simulink model "DEC_DIP_p2014"  (R2013b)
settings: Solver=ode5  StartTime=0.01  StopTime=sim_time  FixedStep=0.01  MaxStep=0.001  RelTol=1e-6  AbsTol=1e-6
undefined symbols (not defined in the file or in its folder): Ankle_Gain, body_mgh, dt_ankle, dt_hip, g, h_COM_L, h_COM_T, Hip_Gain, J_B, J_L, J_T, Kd_A_p, Kd_H_p, Kp_A_p, Kp_H_p, l_L, l_T, m_B, m_L, m_T, mgh_B, mgh_T, pp, th_grav_bs, th_grav_ts, th_vfs, trunk_mgh, wf_grav_bs, wf_grav_ts, wf_T_ext_A, wf_T_ext_H, wf_Trans, wf_vfs
settings Model: ExtModeAutoUpdateStatusClock=off  Creator=thomasmergner  LastModifiedBy=lorenz
settings SolverCC: InitialStep=0.001  AutoInsertRateTranBlk=on
settings DataIOCC: LimitDataPoints=off  SignalLoggingSaveFormat=ModelDataLogs  SaveOutput=off  SignalLogging=off  DSMLogging=off  SaveTime=off  ReturnWorkspaceOutputs=on
settings OptimizationCC: BlockReduction=off  BooleanDataType=off  ExpressionDepthLimit=2147483647  InitFltsAndDblsToZero=on
settings DebuggingCC: SaveWithParameterizedLinksMsg=none  SignalResolutionControl=TryResolveAllWithWarning  SolverPrmCheckMsg=none  InheritedTsInSrcMsg=none  MultiTaskDSMMsg=warning  MultiTaskCondExecSysMsg=none  FcnCallInpInsideContextMsg=UseLocalSettings  StateNameClashWarn=warning
settings HardwareCC: TargetUnknown=on
settings RTWCC: IncludeERTFirstTime=on
settings GRTTargetCC: TargetFcnLib=ansi_tfl_tmw.mat  CombineOutputUpdateFcns=off  GRTInterface=on

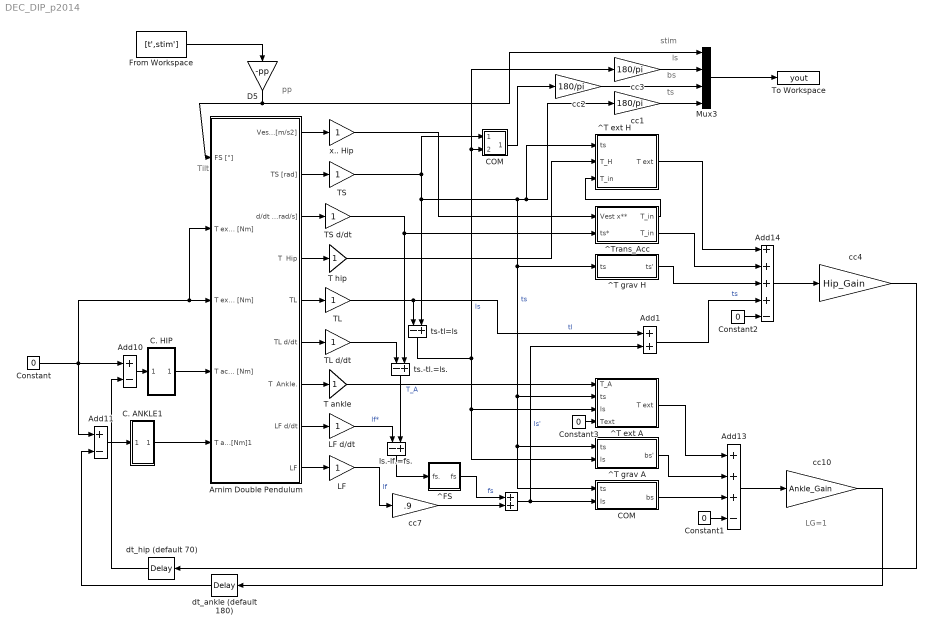
== system DEC_DIP_p2014 ==
  note: Tilt
  note: pp
  note: stim
  note: ls
  note: bs
  note: ts
  note: LG=1
  " " : Sum
  Add1 : Sum
  Add10 : Sum  Inputs=+-
  Add11 : Sum  Inputs=+-
  Add13 : Sum  Inputs=+++-
  Add14 : Sum  Inputs=++++-
  Arnim Double Pendulum : Subsystem
  C. ANKLE1 : Subsystem
  C. HIP : Subsystem
  COM : Subsystem
  "COM " : Subsystem
  Constant{,1..3} (4 alike) : Constant  Value=0
  D5 : Gain  Gain=-pp  SaturateOnIntegerOverflow=on  OutDataTypeStr=Inherit: Same as input  ParamDataTypeStr=Inherit: Same as input
  From Workspace : FromWorkspace  VariableName=[t',stim']
  "LF " : Gain
  LF d/dt : Gain
  Mux3 : Mux
  T ankle : Gain
  T hip : Gain
  TL : Gain
  TL d/dt : Gain
  TS : Gain
  TS d/dt : Gain
  To Workspace : ToWorkspace  VariableName=yout
  ^FS : Subsystem
  ^T ext A : Subsystem
  ^T ext H : Subsystem
  ^T grav A : Subsystem
  ^T grav H : Subsystem
  ^Trans_Acc : Subsystem
  cc1 : Gain  Gain=180/pi
  cc10 : Gain  Gain=Ankle_Gain
  cc2 : Gain  Gain=180/pi
  cc3 : Gain  Gain=180/pi
  cc4 : Gain  Gain=Hip_Gain
  cc7 : Gain  Gain=.9
  dt_ankle (default 180) : TransportDelay  DelayTime=dt_ankle
  dt_hip (default 70) : TransportDelay  DelayTime=dt_hip
  ls.-lf.=fs. : Sum  Inputs=-+
  ts-tl=ls : Sum  Inputs=-+
  ts.-tl.=ls. : Sum  Inputs=-+
  x.. Hip : Gain
  wires:
  Add11/1 -> C. ANKLE1/1(C_)
  Add10/1 -> C. HIP/1("C_   ")
  Arnim Double Pendulum/9(LF) -> "LF "/1
  Arnim Double Pendulum/8(LF d/dt) -> LF d/dt/1
  "LF "/1 -> cc7/1  "lf"
  ls.-lf.=fs./1 -> ^FS/1(fs.)
  TL/1 -> ts-tl=ls/1, Add1/1  "tl"
  Add14/1 -> cc4/1
  ts-tl=ls/1 -> ^T grav A/2(ls), ^T ext A/3(ls), cc3/1, "COM "/2(Is)  "ls"
  Arnim Double Pendulum/4("T  Hip ") -> T hip/1
  TS/1 -> cc1/1, ^T ext H/1(ts), ^T ext A/2(ts), ^T grav A/1(ts), COM/1(ts), ^T grav H/1(ts), ts-tl=ls/2, "COM "/1(ts)  "ts"
  Mux3/1 -> To Workspace/1
  Add13/1 -> cc10/1
  D5/1 -> Arnim Double Pendulum/1(FS [°]), Mux3/1
  From Workspace/1 -> D5/1
  cc4/1 -> dt_hip (default 70)/1
  " "/1 -> COM/2(Is), Add1/2  "ls'"
  cc10/1 -> dt_ankle (default 180)/1
  Arnim Double Pendulum/1(Vest_Acc [m/s2]) -> x.. Hip/1
  x.. Hip/1 -> ^Trans_Acc/1(Vest x**)
  cc3/1 -> Mux3/2
  cc2/1 -> Mux3/3
  cc1/1 -> Mux3/4
  C. HIP/1(Hip) -> Arnim Double Pendulum/4(T act hip [Nm])
  C. ANKLE1/1(" An") -> Arnim Double Pendulum/5(" T act ankle [Nm]1")
  LF d/dt/1 -> ls.-lf.=fs./1  "lf*"
  Arnim Double Pendulum/6(TL d/dt) -> TL d/dt/1
  Arnim Double Pendulum/7(T  Ankle.) -> T ankle/1
  Arnim Double Pendulum/5(TL) -> TL/1
  ts.-tl.=ls./1 -> ls.-lf.=fs./2
  Arnim Double Pendulum/3(d/dt TS[rad/s]) -> TS d/dt/1
  Arnim Double Pendulum/2(TS [rad]) -> TS/1
  TS d/dt/1 -> ts.-tl.=ls./2, ^Trans_Acc/2(ts*)
  TL d/dt/1 -> ts.-tl.=ls./1
  COM/1(bs) -> Add13/3
  T ankle/1 -> ^T ext A/1(T_A)  "T_A"
  ^T grav A/1(bs') -> Add13/2
  ^T grav H/1(ts') -> Add14/3
  T hip/1 -> ^T ext H/2(T_H)
  "COM "/1(bs) -> cc2/1
  dt_ankle (default 180)/1 -> Add11/2
  dt_hip (default 70)/1 -> Add10/2
  ^Trans_Acc/1("T_in ") -> ^T ext H/3(T_in)
  ^FS/1(fs) -> " "/1  "fs"
  cc7/1 -> " "/2
  ^T ext A/1(T ext) -> Add13/1
  Add1/1 -> Add14/4  "ts"
  ^T ext H/1(T ext) -> Add14/1
  ^Trans_Acc/2(T_in) -> Add14/2
  Constant/1 -> Arnim Double Pendulum/2(T ext hip [Nm]), Arnim Double Pendulum/3(T ext ankle [Nm]), Add11/1, Add10/1
  Constant1/1 -> Add13/4
  Constant2/1 -> Add14/5
  Constant3/1 -> ^T ext A/4(Text)

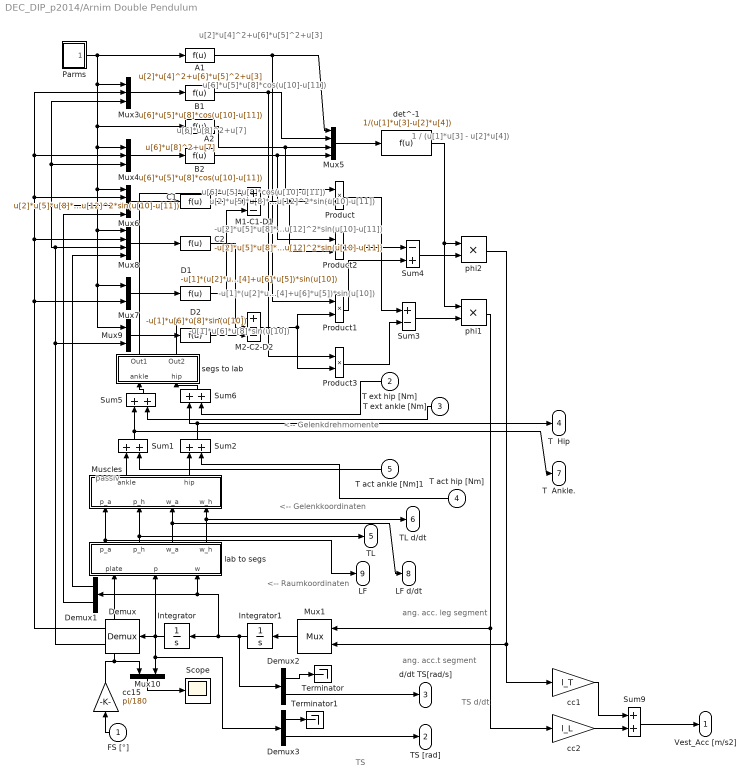
== system DEC_DIP_p2014/Arnim Double Pendulum ==
  note: <-- Gelenkkoordinaten
  note: <-- Gelenkdrehmomente
  note: <-- Raumkoordinaten
  note: ang. acc. leg segment
  note: ang. acc.t segment
  note: u[2]*u[4]^2+u[6]*u[5]^2+u[3]
  note: 1 / (u[1]*u[3] - u[2]*u[4])
  note: u[6]*u[5]*u[8]*cos(u[10]-u[11])
  note: u[6]*u[8]^2+u[7]
  note: u[6]*u[5]*u[8]*cos(u[10]-u[11])
  note: u[2]*u[5]*u[8]*u[12]^2*sin(u[10]-u[11])
  note: -u[2]*u[5]*u[8]*u[12]^2*sin(u[10]-u[11])
  note: -u[1]*(u[2]*u[4]+u[6]*u[5])*sin(u[10])
  note: -u[1]*u[6]*u[8]*sin(u[10])
  note: TS d/dt
  note: TS
  note: passiv
  FS [°] : Inport
  T ext hip [Nm] : Inport  Port=2
  T ext ankle [Nm] : Inport  Port=3
  T act hip [Nm] : Inport  Port=4
  " T act ankle [Nm]1" : Inport  Port=5
  A1 : Fcn  Expr=u[2]*u[4]^2+u[6]*u[5]^2+u[3]
  A2 : Fcn  Expr=u[6]*u[8]^2+u[7]
  B1 : Fcn  Expr=u[6]*u[5]*u[8]*cos(u[10]-u[11])
  B2 : Fcn  Expr=u[6]*u[5]*u[8]*cos(u[10]-u[11])
  C1 : Fcn  Expr=u[2]*u[5]*u[8]*u[12]^2*sin(u[10]-u[11])
  C2 : Fcn  Expr=-u[2]*u[5]*u[8]*u[12]^2*sin(u[10]-u[11])
  D1 : Fcn  Expr=-u[1]*(u[2]*u[4]+u[6]*u[5])*sin(u[10])
  D2 : Fcn  Expr=-u[1]*u[6]*u[8]*sin(u[10])
  Demux{,1..3} (4 alike) : Demux  Outputs=2
  Integrator : Integrator  InitialCondition=[0.0*pi,0.0*pi]
  Integrator1 : Integrator  InitialCondition=[0,0]
  M1-C1-D1 : Sum  Inputs=+--  SaturateOnIntegerOverflow=on  InputSameDT=on  OutDataTypeStr=Inherit: Same as first input
  M2-C2-D2 : Sum  Inputs=+--  SaturateOnIntegerOverflow=on  InputSameDT=on  OutDataTypeStr=Inherit: Same as first input
  Muscles : Subsystem
  Mux{1,7,9..10} (4 alike) : Mux  Inputs=2
  Mux3 : Mux  Inputs=3
  Mux4 : Mux  Inputs=3
  Mux5 : Mux
  Mux6 : Mux
  Mux8 : Mux
  Parms : Subsystem
  Product{,1..3} (4 alike) : Product  SaturateOnIntegerOverflow=on  RndMeth=Zero  InputSameDT=on  OutDataTypeStr=Inherit: Same as first input
  Scope : Scope
      settings: TickLabels=on  YMin=-0.0005  YMax=0.0045
  Sum{1..2,5..6,9} (5 alike) : Sum  SaturateOnIntegerOverflow=on  InputSameDT=on  OutDataTypeStr=Inherit: Same as first input
  Sum3 : Sum  Inputs=+-  SaturateOnIntegerOverflow=on  InputSameDT=on  OutDataTypeStr=Inherit: Same as first input
  Sum4 : Sum  Inputs=-+  SaturateOnIntegerOverflow=on  InputSameDT=on  OutDataTypeStr=Inherit: Same as first input
  Terminator : Terminator
  Terminator1 : Terminator
  cc1 : Gain  Gain=l_T
  cc15 : Gain  Gain=pi/180
  cc2 : Gain  Gain=l_L
  det^-1 : Fcn  Expr=1/(u[1]*u[3]-u[2]*u[4])
  lab to segs : Subsystem
  phi1 : Product  SaturateOnIntegerOverflow=on  RndMeth=Zero  InputSameDT=on  OutDataTypeStr=Inherit: Same as first input
  phi2 : Product  SaturateOnIntegerOverflow=on  RndMeth=Zero  InputSameDT=on  OutDataTypeStr=Inherit: Same as first input
  segs to lab : Subsystem
  Vest_Acc [m/s2] : Outport  InitialOutput=0
  TS [rad] : Outport  Port=2  InitialOutput=0
  d/dt TS[rad/s] : Outport  Port=3  InitialOutput=0
  "T  Hip " : Outport  Port=4  InitialOutput=0
  TL : Outport  Port=5  InitialOutput=0
  TL d/dt : Outport  Port=6  InitialOutput=0
  T  Ankle. : Outport  Port=7  InitialOutput=0
  LF d/dt : Outport  Port=8  InitialOutput=0
  LF : Outport  Port=9  InitialOutput=0
  wires:
  Mux4/1 -> B2/1
  Mux3/1 -> B1/1
  Mux6/1 -> C1/1
  Mux8/1 -> C2/1
  Mux9/1 -> D2/1
  Mux7/1 -> D1/1
  C1/1 -> M1-C1-D1/2
  C2/1 -> M2-C2-D2/2
  D1/1 -> M1-C1-D1/3
  D2/1 -> M2-C2-D2/3
  Parms/1(Out1) -> Mux3/1, A2/1, Mux4/1, Mux9/1, Mux7/1, Mux8/1, Mux6/1, A1/1
  A2/1 -> Mux5/3, Product/1
  M1-C1-D1/1 -> Product/2, Product2/2
  B2/1 -> Mux5/4, Product2/1
  M2-C2-D2/1 -> Product1/2, Product3/2
  A1/1 -> Mux5/1, Product1/1
  B1/1 -> Mux5/2, Product3/1
  Mux5/1 -> det^-1/1
  Product2/1 -> Sum4/1
  Product1/1 -> Sum4/2
  Product3/1 -> Sum3/2
  Product/1 -> Sum3/1
  Sum4/1 -> phi2/2
  Sum3/1 -> phi1/2
  det^-1/1 -> phi2/1, phi1/1
  phi2/1 -> Mux1/2, cc1/1
  Demux/1 -> Mux3/2, Mux4/2, Mux6/2, Mux8/2, Mux7/2
  Demux/2 -> Mux3/3, Mux4/3, Mux6/3, Mux8/3, Mux9/2
  Demux1/1 -> Mux8/4
  Demux1/2 -> Mux6/4
  segs to lab/1(Out1) -> M1-C1-D1/1
  segs to lab/2(Out2) -> M2-C2-D2/1
  Mux1/1 -> Integrator1/1
  Integrator1/1 -> Integrator/1, Demux1/1, lab to segs/3(w), Demux2/1
  Integrator/1 -> Mux10/2, Demux3/1, Demux/1, lab to segs/2(p)
  lab to segs/1(p_a) -> Muscles/1(p_a), LF/1
  lab to segs/2(p_h) -> Muscles/2(p_h), TL/1
  lab to segs/4(w_h) -> Muscles/4(w_h), TL d/dt/1
  lab to segs/3(w_a) -> Muscles/3(w_a), LF d/dt/1
  FS [°]/1 -> cc15/1
  Mux10/1 -> Scope/1
  phi1/1 -> Mux1/1, cc2/1
  " T act ankle [Nm]1"/1 -> Sum1/2
  T act hip [Nm]/1 -> Sum2/2
  Demux2/2 -> d/dt TS[rad/s]/1
  Demux3/2 -> TS [rad]/1
  Sum5/1 -> segs to lab/1(ankle)
  Sum6/1 -> segs to lab/2(hip)
  Sum1/1 -> Sum5/1, T  Ankle./1
  Sum2/1 -> Sum6/1, "T  Hip "/1
  Muscles/1(ankle) -> Sum1/1
  Muscles/2(hip) -> Sum2/1
  cc15/1 -> lab to segs/1(plate), Mux10/1
  T ext hip [Nm]/1 -> Sum6/2
  T ext ankle [Nm]/1 -> Sum5/2
  cc2/1 -> Sum9/2
  Sum9/1 -> Vest_Acc [m/s2]/1
  cc1/1 -> Sum9/1
  Demux2/1 -> Terminator/1
  Demux3/1 -> Terminator1/1

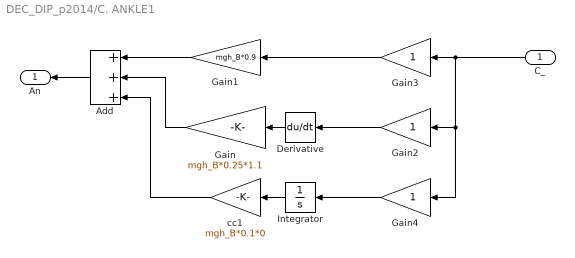
== system DEC_DIP_p2014/C. ANKLE1 ==
  C_ : Inport
  Add : Sum  Inputs=+++
  Derivative : Derivative
  Gain : Gain  Gain=mgh_B*0.25*1.1
  Gain1 : Gain  Gain=mgh_B*0.9
  Gain2 : Gain
  Gain3 : Gain
  Gain4 : Gain
  Integrator : Integrator
  cc1 : Gain  Gain=mgh_B*0.1*0
  " An" : Outport
  wires:
  Derivative/1 -> Gain/1
  Gain/1 -> Add/2
  Gain1/1 -> Add/1
  cc1/1 -> Add/3
  Integrator/1 -> cc1/1
  C_/1 -> Gain2/1, Gain4/1, Gain3/1
  Gain2/1 -> Derivative/1
  Gain3/1 -> Gain1/1
  Gain4/1 -> Integrator/1
  Add/1 -> " An"/1

== system DEC_DIP_p2014/C. HIP ==
  "C_   " : Inport
  Add : Sum  Inputs=+++
  Derivative : Derivative
  Gain : Gain  Gain=mgh_T/4*0.7
  Gain1 : Gain  Gain=mgh_T*0.8
  Gain2 : Gain
  Gain3 : Gain
  Gain4 : Gain
  Integrator : Integrator
  cc2 : Gain  Gain=mgh_T*0.1*0
  Hip : Outport
  wires:
  Add/1 -> Hip/1
  Derivative/1 -> Gain/1
  Gain/1 -> Add/2
  Gain1/1 -> Add/1
  cc2/1 -> Add/3
  Integrator/1 -> cc2/1
  "C_   "/1 -> Gain2/1, Gain3/1, Gain4/1
  Gain2/1 -> Integrator/1
  Gain3/1 -> Derivative/1
  Gain4/1 -> Gain1/1

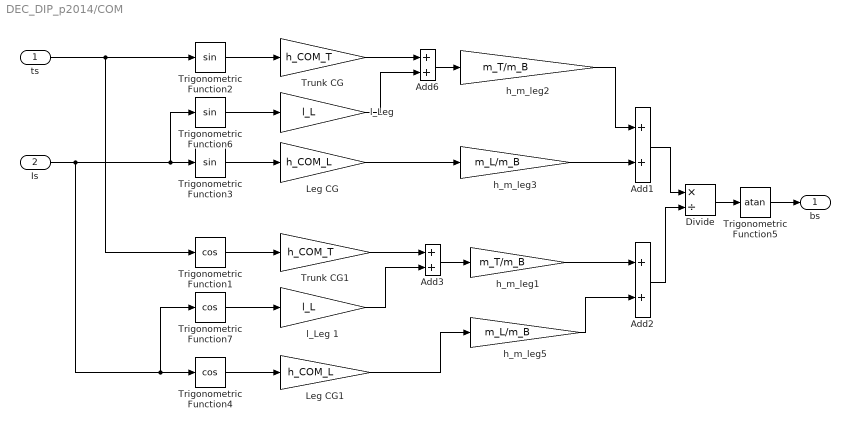
== system DEC_DIP_p2014/COM ==
  ts : Inport
  Is : Inport  Port=2
  Add{1..3,6} (4 alike) : Sum
  Divide : Product  Inputs=*/
  Leg CG : Gain  Gain=h_COM_L
  Leg CG1 : Gain  Gain=h_COM_L
  Trigonometric Function1 : Trigonometry  Operator=cos
  Trigonometric Function2 : Trigonometry
  Trigonometric Function3 : Trigonometry
  Trigonometric Function4 : Trigonometry  Operator=cos
  Trigonometric Function5 : Trigonometry  Operator=atan
  Trigonometric Function6 : Trigonometry
  Trigonometric Function7 : Trigonometry  Operator=cos
  Trunk CG : Gain  Gain=h_COM_T
  Trunk CG1 : Gain  Gain=h_COM_T
  h_m_leg1 : Gain  Gain=m_T/m_B
  h_m_leg2 : Gain  Gain=m_T/m_B
  h_m_leg3 : Gain  Gain=m_L/m_B
  h_m_leg5 : Gain  Gain=m_L/m_B
  "l_Leg " : Gain  Gain=l_L
  l_Leg 1 : Gain  Gain=l_L
  bs : Outport
  wires:
  ts/1 -> Trigonometric Function1/1, Trigonometric Function2/1
  Trigonometric Function2/1 -> Trunk CG/1
  Trigonometric Function3/1 -> Leg CG/1
  Is/1 -> Trigonometric Function3/1, Trigonometric Function6/1, Trigonometric Function4/1, Trigonometric Function7/1
  Trunk CG/1 -> Add6/1
  h_m_leg3/1 -> Add1/2
  Add6/1 -> h_m_leg2/1
  "l_Leg "/1 -> Add6/2
  Trigonometric Function1/1 -> Trunk CG1/1
  Trigonometric Function4/1 -> Leg CG1/1
  Trunk CG1/1 -> Add3/1
  Leg CG1/1 -> h_m_leg5/1
  h_m_leg1/1 -> Add2/1
  h_m_leg5/1 -> Add2/2
  Add3/1 -> h_m_leg1/1
  Add1/1 -> Divide/1
  Divide/1 -> Trigonometric Function5/1
  Trigonometric Function5/1 -> bs/1
  Leg CG/1 -> h_m_leg3/1
  h_m_leg2/1 -> Add1/1
  Add2/1 -> Divide/2
  Trigonometric Function6/1 -> "l_Leg "/1
  Trigonometric Function7/1 -> l_Leg 1/1
  l_Leg 1/1 -> Add3/2

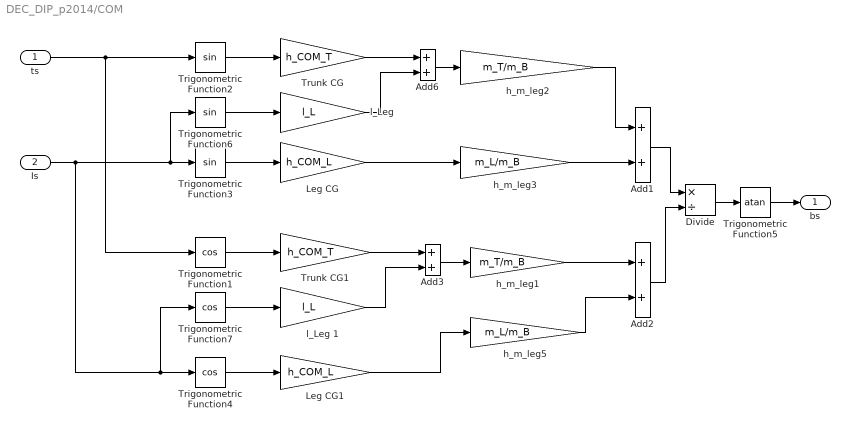
== system DEC_DIP_p2014/COM  ==
  ts : Inport
  Is : Inport  Port=2
  Add{1..3,6} (4 alike) : Sum
  Divide : Product  Inputs=*/
  Leg CG : Gain  Gain=h_COM_L
  Leg CG1 : Gain  Gain=h_COM_L
  Trigonometric Function1 : Trigonometry  Operator=cos
  Trigonometric Function2 : Trigonometry
  Trigonometric Function3 : Trigonometry
  Trigonometric Function4 : Trigonometry  Operator=cos
  Trigonometric Function5 : Trigonometry  Operator=atan
  Trigonometric Function6 : Trigonometry
  Trigonometric Function7 : Trigonometry  Operator=cos
  Trunk CG : Gain  Gain=h_COM_T
  Trunk CG1 : Gain  Gain=h_COM_T
  h_m_leg1 : Gain  Gain=m_T/m_B
  h_m_leg2 : Gain  Gain=m_T/m_B
  h_m_leg3 : Gain  Gain=m_L/m_B
  h_m_leg5 : Gain  Gain=m_L/m_B
  "l_Leg " : Gain  Gain=l_L
  l_Leg 1 : Gain  Gain=l_L
  bs : Outport
  wires:
  l_Leg 1/1 -> Add3/2
  Trigonometric Function7/1 -> l_Leg 1/1
  Trigonometric Function6/1 -> "l_Leg "/1
  Add2/1 -> Divide/2
  h_m_leg2/1 -> Add1/1
  Leg CG/1 -> h_m_leg3/1
  Trigonometric Function5/1 -> bs/1
  Divide/1 -> Trigonometric Function5/1
  Add1/1 -> Divide/1
  Add3/1 -> h_m_leg1/1
  h_m_leg5/1 -> Add2/2
  h_m_leg1/1 -> Add2/1
  Leg CG1/1 -> h_m_leg5/1
  Trunk CG1/1 -> Add3/1
  Trigonometric Function4/1 -> Leg CG1/1
  Trigonometric Function1/1 -> Trunk CG1/1
  "l_Leg "/1 -> Add6/2
  Add6/1 -> h_m_leg2/1
  h_m_leg3/1 -> Add1/2
  Trunk CG/1 -> Add6/1
  Is/1 -> Trigonometric Function7/1, Trigonometric Function4/1, Trigonometric Function6/1, Trigonometric Function3/1
  Trigonometric Function3/1 -> Leg CG/1
  Trigonometric Function2/1 -> Trunk CG/1
  ts/1 -> Trigonometric Function2/1, Trigonometric Function1/1

== system DEC_DIP_p2014/^FS ==
  fs. : Inport
  D1 : Gain  Gain=wf_vfs  SaturateOnIntegerOverflow=on  OutDataTypeStr=Inherit: Same as input  ParamDataTypeStr=Inherit: Same as input
  Integrator : Integrator
  th_vfs : DeadZone  LowerValue=-th_vfs  UpperValue=th_vfs  SaturateOnIntegerOverflow=on
  fs : Outport
  wires:
  fs./1 -> th_vfs/1
  Integrator/1 -> fs/1
  D1/1 -> Integrator/1
  th_vfs/1 -> D1/1

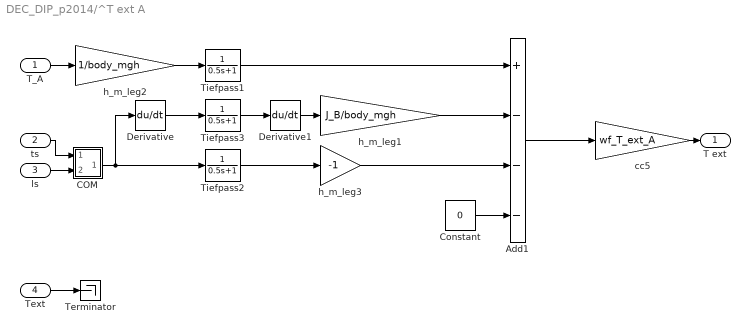
== system DEC_DIP_p2014/^T ext A ==
  T_A : Inport
  ts : Inport  Port=2
  ls : Inport  Port=3
  Text : Inport  Port=4
  Add1 : Sum  Inputs=+---
  COM : Subsystem
  Constant : Constant  Value=0
  Derivative : Derivative
  Derivative1 : Derivative
  Terminator : Terminator
  Tiefpass1 : TransferFcn  Denominator=[0.5 1]
  Tiefpass2 : TransferFcn  Denominator=[0.5 1]
  Tiefpass3 : TransferFcn  Denominator=[0.5 1]
  cc5 : Gain  Gain=wf_T_ext_A
  h_m_leg1 : Gain  Gain=J_B/body_mgh
  h_m_leg2 : Gain  Gain=1/body_mgh
  h_m_leg3 : Gain  Gain=-1
  T ext : Outport
  wires:
  cc5/1 -> T ext/1
  ls/1 -> COM/2(Is)
  ts/1 -> COM/1(ts)
  T_A/1 -> h_m_leg2/1
  Add1/1 -> cc5/1
  COM/1(bs) -> Tiefpass2/1, Derivative/1
  h_m_leg2/1 -> Tiefpass1/1
  Tiefpass1/1 -> Add1/1
  Tiefpass2/1 -> h_m_leg3/1
  Derivative/1 -> Tiefpass3/1
  Tiefpass3/1 -> Derivative1/1
  Derivative1/1 -> h_m_leg1/1
  h_m_leg1/1 -> Add1/2
  Text/1 -> Terminator/1
  h_m_leg3/1 -> Add1/3
  Constant/1 -> Add1/4

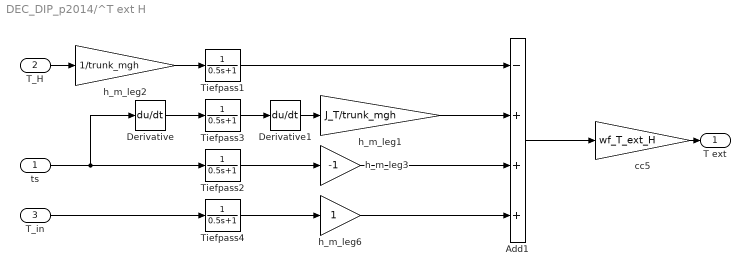
== system DEC_DIP_p2014/^T ext H ==
  ts : Inport
  T_H : Inport  Port=2
  T_in : Inport  Port=3
  Add1 : Sum  Inputs=-+++
  Derivative : Derivative
  Derivative1 : Derivative
  Tiefpass{1..4} (4 alike) : TransferFcn  Denominator=[0.5 1]
  cc5 : Gain  Gain=wf_T_ext_H
  h_m_leg1 : Gain  Gain=J_T/trunk_mgh
  h_m_leg2 : Gain  Gain=1/trunk_mgh
  h_m_leg3 : Gain  Gain=-1
  h_m_leg6 : Gain
  T ext : Outport
  wires:
  h_m_leg3/1 -> Add1/3
  h_m_leg1/1 -> Add1/2
  Derivative1/1 -> h_m_leg1/1
  Tiefpass3/1 -> Derivative1/1
  Derivative/1 -> Tiefpass3/1
  Tiefpass2/1 -> h_m_leg3/1
  Tiefpass1/1 -> Add1/1
  h_m_leg2/1 -> Tiefpass1/1
  Add1/1 -> cc5/1
  T_H/1 -> h_m_leg2/1
  cc5/1 -> T ext/1
  ts/1 -> Tiefpass2/1, Derivative/1
  T_in/1 -> Tiefpass4/1
  Tiefpass4/1 -> h_m_leg6/1
  h_m_leg6/1 -> Add1/4

== system DEC_DIP_p2014/^T grav A ==
  ts : Inport
  ls : Inport  Port=2
  Add1 : Sum
  COM : Subsystem
  Tiefpass2 : TransferFcn  Numerator=[15]  Denominator=[15 1]
  cc1 : Gain  Gain=0.2
  cc5 : Gain  Gain=wf_grav_bs
  th_grav_bs : DeadZone  LowerValue=-th_grav_bs  UpperValue=th_grav_bs  SaturateOnIntegerOverflow=on
  bs' : Outport
  wires:
  COM/1(bs) -> th_grav_bs/1
  th_grav_bs/1 -> cc5/1, Tiefpass2/1
  ts/1 -> COM/1(ts)
  ls/1 -> COM/2(Is)
  Add1/1 -> bs'/1
  cc5/1 -> Add1/2
  Tiefpass2/1 -> cc1/1
  cc1/1 -> Add1/1

== system DEC_DIP_p2014/^T grav H ==
  ts : Inport
  0.16 : DeadZone  LowerValue=-th_grav_ts  UpperValue=th_grav_ts  SaturateOnIntegerOverflow=on
  0.8 : Gain  Gain=wf_grav_ts
  Add1 : Sum
  Tiefpass2 : TransferFcn  Numerator=[15]  Denominator=[15 1]
  cc1 : Gain  Gain=0.2
  ts' : Outport
  wires:
  ts/1 -> 0.16/1
  0.16/1 -> 0.8/1, Tiefpass2/1
  Tiefpass2/1 -> cc1/1
  0.8/1 -> Add1/1
  Add1/1 -> ts'/1
  cc1/1 -> Add1/2

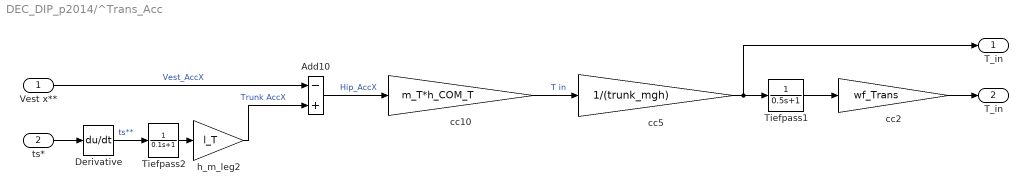
== system DEC_DIP_p2014/^Trans_Acc ==
  Vest x** : Inport
  ts* : Inport  Port=2
  Add10 : Sum  Inputs=-+
  Derivative : Derivative
  Tiefpass1 : TransferFcn  Denominator=[0.5 1]
  Tiefpass2 : TransferFcn  Denominator=[0.1 1]
  cc10 : Gain  Gain=m_T*h_COM_T
  cc2 : Gain  Gain=wf_Trans
  cc5 : Gain  Gain=1/(trunk_mgh)
  h_m_leg2 : Gain  Gain=l_T
  "T_in " : Outport
  T_in : Outport  Port=2
  wires:
  cc10/1 -> cc5/1  "T in"
  cc5/1 -> Tiefpass1/1, "T_in "/1
  Vest x**/1 -> Add10/1  "Vest_AccX"
  cc2/1 -> T_in/1
  Add10/1 -> cc10/1  "Hip_AccX"
  ts*/1 -> Derivative/1
  Derivative/1 -> Tiefpass2/1  "ts**"
  h_m_leg2/1 -> Add10/2  "Trunk AccX"
  Tiefpass2/1 -> h_m_leg2/1
  Tiefpass1/1 -> cc2/1

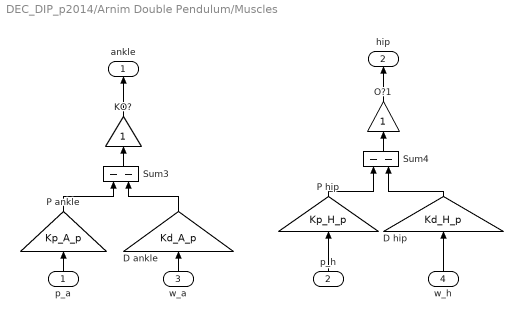
== system DEC_DIP_p2014/Arnim Double Pendulum/Muscles ==
  p_a : Inport
  p_h : Inport  Port=2
  w_a : Inport  Port=3
  w_h : Inport  Port=4
  D ankle : Gain  Gain=Kd_A_p  SaturateOnIntegerOverflow=on  OutDataTypeStr=Inherit: Same as input  ParamDataTypeStr=Inherit: Same as input
  D hip : Gain  Gain=Kd_H_p  SaturateOnIntegerOverflow=on  OutDataTypeStr=Inherit: Same as input  ParamDataTypeStr=Inherit: Same as input
  KO? : Gain  SaturateOnIntegerOverflow=on  OutDataTypeStr=Inherit: Same as input  ParamDataTypeStr=Inherit: Same as input
  O?1 : Gain  SaturateOnIntegerOverflow=on  OutDataTypeStr=Inherit: Same as input  ParamDataTypeStr=Inherit: Same as input
  P ankle : Gain  Gain=Kp_A_p  SaturateOnIntegerOverflow=on  OutDataTypeStr=Inherit: Same as input  ParamDataTypeStr=Inherit: Same as input
  P hip : Gain  Gain=Kp_H_p  SaturateOnIntegerOverflow=on  OutDataTypeStr=Inherit: Same as input  ParamDataTypeStr=Inherit: Same as input
  Sum3 : Sum  Inputs=--  SaturateOnIntegerOverflow=on  InputSameDT=on  OutDataTypeStr=Inherit: Same as first input
  Sum4 : Sum  Inputs=--  SaturateOnIntegerOverflow=on  InputSameDT=on  OutDataTypeStr=Inherit: Same as first input
  ankle : Outport  InitialOutput=0
  hip : Outport  Port=2  InitialOutput=0
  wires:
  P ankle/1 -> Sum3/1
  D ankle/1 -> Sum3/2
  p_a/1 -> P ankle/1
  w_a/1 -> D ankle/1
  P hip/1 -> Sum4/1
  p_h/1 -> P hip/1
  w_h/1 -> D hip/1
  Sum4/1 -> O?1/1
  D hip/1 -> Sum4/2
  O?1/1 -> hip/1
  KO?/1 -> ankle/1
  Sum3/1 -> KO?/1

== system DEC_DIP_p2014/Arnim Double Pendulum/Parms ==
  J_L : Constant  Value=J_L
  J_T : Constant  Value=J_T
  Mux : Mux  Inputs=9
  g : Constant  Value=g
  h_m_leg : Constant  Value=h_COM_L
  h_m_trunk : Constant  Value=h_COM_T
  l_leg : Constant  Value=l_L
  l_trunk : Constant  Value=l_T
  m_leg : Constant  Value=m_L
  m_trunk : Constant  Value=m_T
  Out1 : Outport  InitialOutput=0
  wires:
  l_trunk/1 -> Mux/9
  h_m_trunk/1 -> Mux/8
  J_T/1 -> Mux/7
  l_leg/1 -> Mux/5
  h_m_leg/1 -> Mux/4
  J_L/1 -> Mux/3
  m_leg/1 -> Mux/2
  m_trunk/1 -> Mux/6
  Mux/1 -> Out1/1
  g/1 -> Mux/1

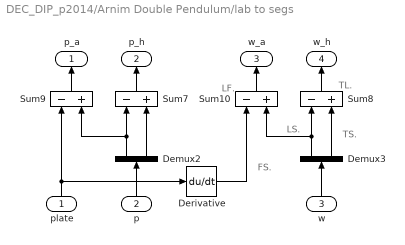
== system DEC_DIP_p2014/Arnim Double Pendulum/lab to segs ==
  note: FS.
  note: LS.
  note: LF.
  note: TL.
  note: TS.
  plate : Inport
  p : Inport  Port=2
  w : Inport  Port=3
  Demux2 : Demux  Outputs=2
  Demux3 : Demux  Outputs=2
  Derivative : Derivative
  Sum{7..10} (4 alike) : Sum  Inputs=-+  SaturateOnIntegerOverflow=on  InputSameDT=on  OutDataTypeStr=Inherit: Same as first input
  p_a : Outport  InitialOutput=0
  p_h : Outport  Port=2  InitialOutput=0
  w_a : Outport  Port=3  InitialOutput=0
  w_h : Outport  Port=4  InitialOutput=0
  wires:
  p/1 -> Demux2/1
  Demux2/2 -> Sum7/2
  Sum7/1 -> p_h/1
  Demux2/1 -> Sum7/1, Sum9/2
  Sum9/1 -> p_a/1
  plate/1 -> Sum9/1, Derivative/1
  w/1 -> Demux3/1
  Demux3/2 -> Sum8/2
  Sum8/1 -> w_h/1
  Sum10/1 -> w_a/1
  Demux3/1 -> Sum8/1, Sum10/2
  Derivative/1 -> Sum10/1

== system DEC_DIP_p2014/Arnim Double Pendulum/segs to lab ==
  ankle : Inport
  hip : Inport  Port=2
  Sum5 : Sum  Inputs=+-  SaturateOnIntegerOverflow=on  InputSameDT=on  OutDataTypeStr=Inherit: Same as first input
  Out1 : Outport  InitialOutput=0
  Out2 : Outport  Port=2  InitialOutput=0
  wires:
  Sum5/1 -> Out1/1
  ankle/1 -> Sum5/1
  hip/1 -> Out2/1, Sum5/2

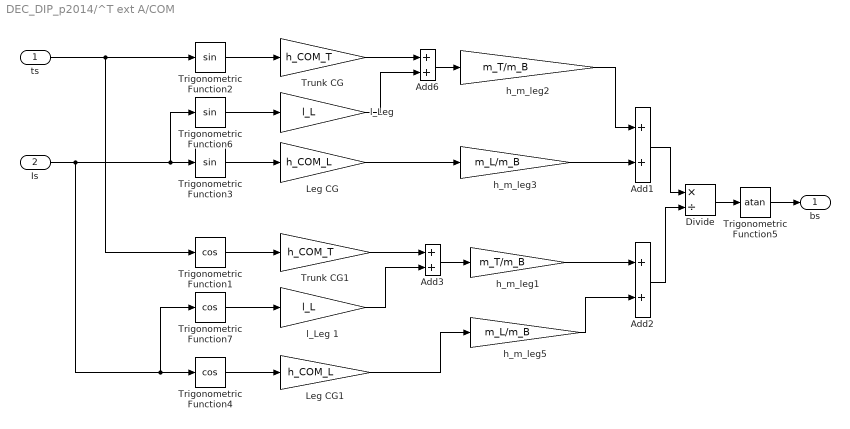
== system DEC_DIP_p2014/^T ext A/COM ==
  ts : Inport
  Is : Inport  Port=2
  Add{1..3,6} (4 alike) : Sum
  Divide : Product  Inputs=*/
  Leg CG : Gain  Gain=h_COM_L
  Leg CG1 : Gain  Gain=h_COM_L
  Trigonometric Function1 : Trigonometry  Operator=cos
  Trigonometric Function2 : Trigonometry
  Trigonometric Function3 : Trigonometry
  Trigonometric Function4 : Trigonometry  Operator=cos
  Trigonometric Function5 : Trigonometry  Operator=atan
  Trigonometric Function6 : Trigonometry
  Trigonometric Function7 : Trigonometry  Operator=cos
  Trunk CG : Gain  Gain=h_COM_T
  Trunk CG1 : Gain  Gain=h_COM_T
  h_m_leg1 : Gain  Gain=m_T/m_B
  h_m_leg2 : Gain  Gain=m_T/m_B
  h_m_leg3 : Gain  Gain=m_L/m_B
  h_m_leg5 : Gain  Gain=m_L/m_B
  "l_Leg " : Gain  Gain=l_L
  l_Leg 1 : Gain  Gain=l_L
  bs : Outport
  wires:
  ts/1 -> Trigonometric Function1/1, Trigonometric Function2/1
  Trigonometric Function2/1 -> Trunk CG/1
  Trigonometric Function3/1 -> Leg CG/1
  Is/1 -> Trigonometric Function3/1, Trigonometric Function6/1, Trigonometric Function4/1, Trigonometric Function7/1
  Trunk CG/1 -> Add6/1
  h_m_leg3/1 -> Add1/2
  Add6/1 -> h_m_leg2/1
  "l_Leg "/1 -> Add6/2
  Trigonometric Function1/1 -> Trunk CG1/1
  Trigonometric Function4/1 -> Leg CG1/1
  Trunk CG1/1 -> Add3/1
  Leg CG1/1 -> h_m_leg5/1
  h_m_leg1/1 -> Add2/1
  h_m_leg5/1 -> Add2/2
  Add3/1 -> h_m_leg1/1
  Add1/1 -> Divide/1
  Divide/1 -> Trigonometric Function5/1
  Trigonometric Function5/1 -> bs/1
  Leg CG/1 -> h_m_leg3/1
  h_m_leg2/1 -> Add1/1
  Add2/1 -> Divide/2
  Trigonometric Function6/1 -> "l_Leg "/1
  Trigonometric Function7/1 -> l_Leg 1/1
  l_Leg 1/1 -> Add3/2

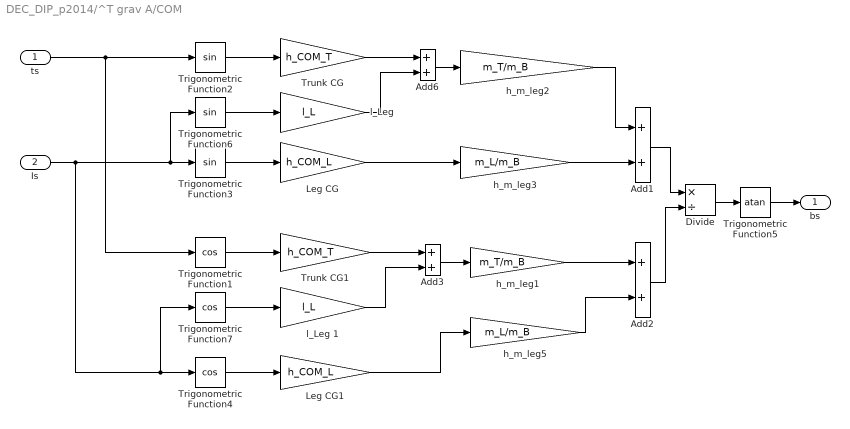
== system DEC_DIP_p2014/^T grav A/COM ==
  ts : Inport
  Is : Inport  Port=2
  Add{1..3,6} (4 alike) : Sum
  Divide : Product  Inputs=*/
  Leg CG : Gain  Gain=h_COM_L
  Leg CG1 : Gain  Gain=h_COM_L
  Trigonometric Function1 : Trigonometry  Operator=cos
  Trigonometric Function2 : Trigonometry
  Trigonometric Function3 : Trigonometry
  Trigonometric Function4 : Trigonometry  Operator=cos
  Trigonometric Function5 : Trigonometry  Operator=atan
  Trigonometric Function6 : Trigonometry
  Trigonometric Function7 : Trigonometry  Operator=cos
  Trunk CG : Gain  Gain=h_COM_T
  Trunk CG1 : Gain  Gain=h_COM_T
  h_m_leg1 : Gain  Gain=m_T/m_B
  h_m_leg2 : Gain  Gain=m_T/m_B
  h_m_leg3 : Gain  Gain=m_L/m_B
  h_m_leg5 : Gain  Gain=m_L/m_B
  "l_Leg " : Gain  Gain=l_L
  l_Leg 1 : Gain  Gain=l_L
  bs : Outport
  wires:
  l_Leg 1/1 -> Add3/2
  Trigonometric Function7/1 -> l_Leg 1/1
  Trigonometric Function6/1 -> "l_Leg "/1
  Add2/1 -> Divide/2
  h_m_leg2/1 -> Add1/1
  Leg CG/1 -> h_m_leg3/1
  Trigonometric Function5/1 -> bs/1
  Divide/1 -> Trigonometric Function5/1
  Add1/1 -> Divide/1
  Add3/1 -> h_m_leg1/1
  h_m_leg5/1 -> Add2/2
  h_m_leg1/1 -> Add2/1
  Leg CG1/1 -> h_m_leg5/1
  Trunk CG1/1 -> Add3/1
  Trigonometric Function4/1 -> Leg CG1/1
  Trigonometric Function1/1 -> Trunk CG1/1
  "l_Leg "/1 -> Add6/2
  Add6/1 -> h_m_leg2/1
  h_m_leg3/1 -> Add1/2
  Trunk CG/1 -> Add6/1
  Is/1 -> Trigonometric Function7/1, Trigonometric Function4/1, Trigonometric Function6/1, Trigonometric Function3/1
  Trigonometric Function3/1 -> Leg CG/1
  Trigonometric Function2/1 -> Trunk CG/1
  ts/1 -> Trigonometric Function2/1, Trigonometric Function1/1
